simulink model "Furuta_Pendulum"  (R2024b)
settings: Solver=VariableStepAuto  StartTime=0.0  StopTime=10  RelTol=1e-3
settings Model: Creator=sahilpandey  LastModifiedBy=sahilpandey

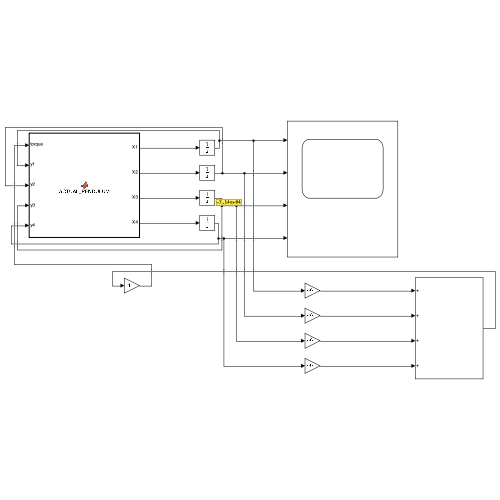
[thumbnail: Simulink's stored preview of the top-level diagram]
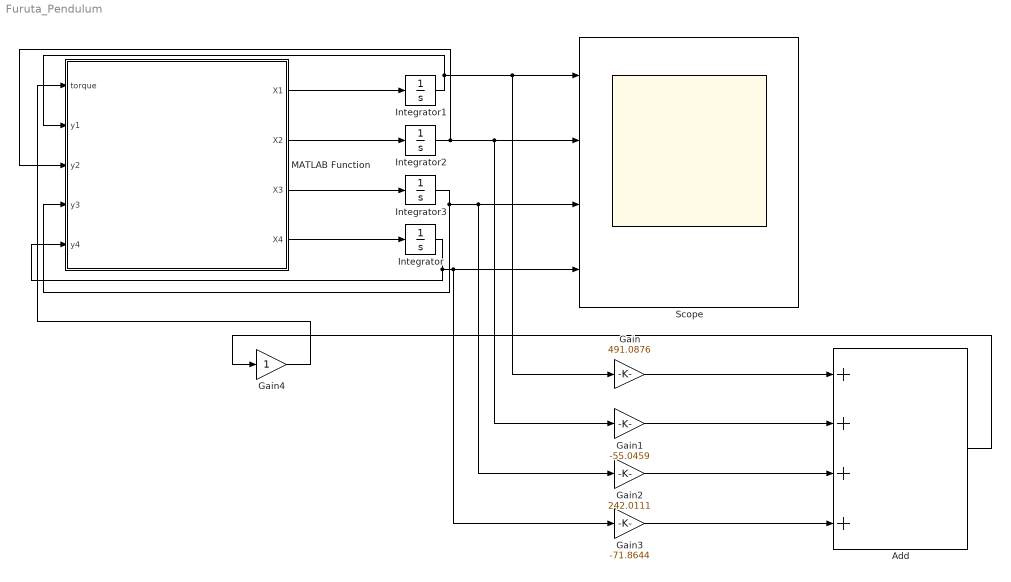
== system Furuta_Pendulum ==
  Add : Sum  Inputs=++++
  Gain : Gain  Gain=491.0876
  Gain1 : Gain  Gain=-55.0459
  Gain2 : Gain  Gain=242.0111
  Gain3 : Gain  Gain=-71.8644
  Gain4 : Gain
  Integrator : Integrator
  Integrator1 : Integrator  InitialCondition=pi/10
  Integrator2 : Integrator  InitialCondition=pi/2
  Integrator3 : Integrator
  MATLAB Function : MATLAB Function  TreatAsAtomicUnit=on
  Scope : Scope  NumInputPorts=4
  wires:
  MATLAB Function/1(X1) -> Integrator1/1
  MATLAB Function/2(X2) -> Integrator2/1
  MATLAB Function/3(X3) -> Integrator3/1
  MATLAB Function/4(X4) -> Integrator/1
  Integrator1/1 -> MATLAB Function/2(y1), Gain/1, Scope/1
  Integrator2/1 -> MATLAB Function/3(y2), Gain1/1, Scope/2
  Integrator3/1 -> MATLAB Function/4(y3), Gain2/1, Scope/3
  Integrator/1 -> MATLAB Function/5(y4), Scope/4, Gain3/1
  Gain4/1 -> MATLAB Function/1(torque)
  Gain/1 -> Add/1
  Gain1/1 -> Add/2
  Gain2/1 -> Add/3
  Gain3/1 -> Add/4
  Add/1 -> Gain4/1

== matlab function Furuta_Pendulum/MATLAB Function ==
  data: torque input; X1 output; y1 input; y2 input; y3 input; y4 input; X2 output; X3 output; X4 output

function [X1,X2,X3,X4]=ACTUAL_PENDULUM(torque,y1,y2,y3,y4)
    
    mp=1; % mass of pendulum
    d=0.5; %distance of COM of pendulum from piviot
    Ip=1; %MOI of pendulum about COM;
    Bp=0; %damping coefficient of pendulum
    Br=0; %damping coefficient of arm
    l=1; %length of arm
    Ir=1; %MOI of arm wrt piviot
    g=9.81; %gravity
    
    A=(mp*l*l + mp*d*d*cos(y1) + Ir);
    B=mp*l*d*cos(y1);
    C=(mp*y3*y4*d*d*sin(2*y1)) + mp*d*l*sin(y1)*y3*y3;
    D=(mp*d*(d/2)*sin(2*(y1))) + mp*g*d*sin(y1);
    E=mp*d*d+Ip;
    X1= y3; %theta
    X2= y4; %phi
    X3= ((torque - Br*y4)*B - (Bp*y3)*A - (C*B) + (D*A)) / (E*A) ;    %theta.
    X4= ((torque-Br*y4) - C + B * X3)/A ;     %phi.

end
